simulink model "Check_LQRI_sim"  (R2017b)
settings: Solver=VariableStepAuto  StartTime=0.0  StopTime=10.0  RelTol=1e-3
values from neighbouring files (symbols this model uses):
  A = [0 v0;0 0]    [Check_Discretization.m]
  B = [0;1]    [Check_Discretization.m]
  C = diag([1 1])    [Check_Discretization.m]
  D = [0;0]    [Check_Discretization.m]
  Ts = 0.1    [Check_Discretization.m]
undefined symbols (not defined in the file or in its folder): Ad, Bd, Cd, Dd, sigbuilder_block
settings Model: Creator=lukas  LastModifiedBy=lukas

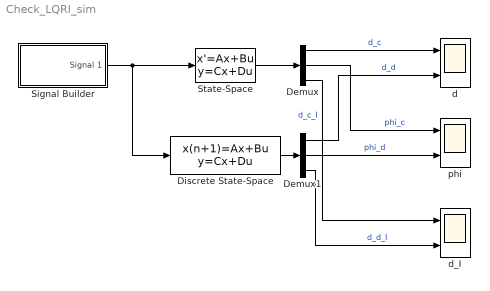
== system Check_LQRI_sim ==
  Demux : Demux  Outputs=3
  Demux1 : Demux  Outputs=3
  Discrete State-Space : DiscreteStateSpace  A=Ad  B=Bd  C=Cd  D=Dd  SampleTime=Ts
  Signal Builder : Subsystem  Tag=STV Subsys  LoadFcn=sigbuilder_block('load');  StartFcn=sigbuilder_block('start');  StopFcn=sigbuilder_block('stop');  ClipboardFcn=sigbuilder_block('clipboard');  mask(Sigbuilder block){tuvar=[0:10]}
      mask help: Simulink:masks:SigbuilderBlock_MD
      mask init:
      | if ~strcmp(get_param(bdroot(gcbh),'SimulationStatus'),'stopped') tuvar = sigbuilder_block('maskInit'); end
      settings: CopyFcn=sigbuilder_block('copy');  DeleteFcn=sigbuilder_block('delete');  ModelCloseFcn=sigbuilder_block('modelClose');  PreSaveFcn=sigbuilder_block('preSave');  PauseFcn=sigbuilder_block('pause');  ContinueFcn=sigbuilder_block('continue');  NameChangeFcn=sigbuilder_block('namechange');  OpenFcn=sigbuilder_block('open',[437.6 199.2 550.4 400 ]);  CloseFcn=sigbuilder_block('close');
      mask Display: plot(0, 0, 100, 100,[2, 2, 32, 32, 2], [68, 8, 8, 68, 68],[32, 2], [38, 38], [32, 19, 2],[53, 60, 44], [32, 17, 17, 2],[16, 16, 31, 31]);txt = getActiveGroup(gcbh);text(2, 100, txt,'verticalAlignment', 'top');
  State-Space : StateSpace  A=A  B=B  C=C  D=D  InitialCondition=0
  d : Scope  NumInputPorts=2
  d_I : Scope  NumInputPorts=2
  phi : Scope  NumInputPorts=2
  wires:
  Demux1/1 -> d/2  "d_d"
  Demux/2 -> phi/1  "phi_c"
  State-Space/1 -> Demux/1
  Demux1/2 -> phi/2  "phi_d"
  Discrete State-Space/1 -> Demux1/1
  Signal Builder/1(Signal 1) -> Discrete State-Space/1, State-Space/1
  Demux/1 -> d/1  "d_c"
  Demux/3 -> d_I/1  "d_c_I"
  Demux1/3 -> d_I/2  "d_d_I"

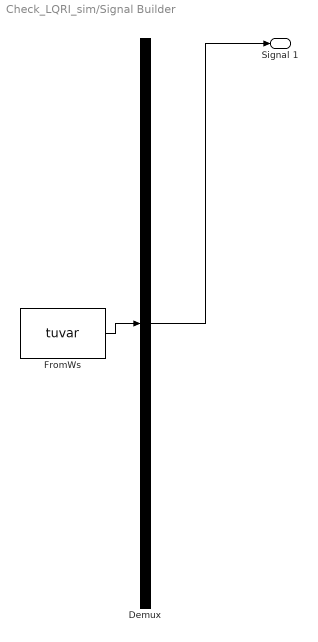
== system Check_LQRI_sim/Signal Builder ==
  Demux : Demux  Tag=STV Demux  Outputs=1
  FromWs : FromWorkspace  Tag=STV FromWs  VariableName=tuvar  SampleTime=0
      SigBuilderData=|
      | common.afterFinalStr = 'Extrapolate'
      | common.sampleTime = 0
      | dataSet.timeRange = [0 10]
      | dataSet.name = 'Group 1'
      | sbobj.Groups.Name = 'Group 1'
      | sbobj.Groups.Signals.Name = 'Signal 1'
      | sbobj.Groups.Signals.XData = [0 2 2 6 6 10]
      | sbobj.Groups.Signals.YData = [0 0 1 1 -1 -1]
  Signal 1 : Outport  Tag=STV Outport
  wires:
  Demux/1 -> Signal 1/1
  FromWs/1 -> Demux/1
